simulink model "power_microgrid_v5_battery"  (R2018b)
settings: Solver=ode23tb  StartTime=0.0  StopTime=24*60*60  FixedStep=1/(1000)  MaxStep=60  RelTol=1e-4
PreLoadFcn:
  | load('solar_load_data_24h.mat')
PostLoadFcn:
  | data = xlsread('Domestic_data_all_x3','Sheet1');
  | breakpoints1 = data(2:end,1)'
  | breakpoints2 = data(1,2:end)
  | table_data = data(2:end,2:end)
values from neighbouring files (symbols this model uses):
  SPD_1min = [0 0 0 0 0 0 0 0 0 0 0 0 ... (1441 elements, 1441x1)]    [default_PV_data.mat]
  SPT_1min = [0 60 120 180 240 300 360 420 480 540 600 660 ... (1441 elements, 1441x1)]    [default_PV_data.mat]
libraries: powerlib x155
(part 1 of 5)
Description:
  | Copyright 2008-2018 The MathWorks, Inc.
settings Model: ModifiedByFormat=SPS  ExtModeTrigMode=oneshot  ExtModeArmWhenConnect=off  Creator=MathWorks  LastModifiedBy=SPS
settings SolverCC: InitialStep=1e-4  ZeroCrossAlgorithm=Adaptive
settings DataIOCC: SaveFormat=Array  SignalLoggingSaveFormat=ModelDataLogs  SaveOutput=off  SaveTime=off  SignalLoggingName=sigsOut
settings OptimizationCC: BooleanDataType=off  ExpressionDepthLimit=2147483647  InitFltsAndDblsToZero=on  LifeSpan=inf
settings DebuggingCC: AlgebraicLoopMsg=none  SaveWithParameterizedLinksMsg=none  UnderspecifiedInitializationDetection=Classic  MergeDetectMultiDrivingBlocksExec=none  SignalResolutionControl=TryResolveAllWithWarning  MultiTaskDSMMsg=warning  MultiTaskCondExecSysMsg=none  FcnCallInpInsideContextMsg=warning  AllowSymbolicDim=off  StateNameClashWarn=warning  SFUnexpectedBacktrackingDiag=warning  SFNoUnconditionalDefaultTransitionDiag=warning  SFExecutionAtInitializationDiag=none
settings HardwareCC: ProdBitPerPointer=32  ProdBitPerSizeT=32  ProdBitPerPtrDiffT=32  ProdLargestAtomicFloat=None  ProdIntDivRoundTo=Undefined  ProdEndianess=Unspecified  ProdWordSize=32  ProdHWDeviceType=32-bit Generic  TargetUnknown=on
settings ModelReferenceCC: PropagateSignalLabelsOutOfModel=off
settings SFSimCC: SimUseLocalCustomCode=off
settings RTWCC: Description=Generic Real-Time Target  RTWUseLocalCustomCode=off
settings CodeAppCC: StateflowObjectComments=on
settings GRTTargetCC: TargetFcnLib=ansi_tfl_tmw.mat  TargetLangStandard=C89/C90 (ANSI)  GeneratePreprocessorConditionals=Disable all  CombineOutputUpdateFcns=off  GRTInterface=on
settings ConfigComp: CovMetricSettings=dw  CovHtmlReporting=on  CovSaveCumulativeToWorkspaceVar=on  CovSaveSingleToWorkspaceVar=on  CovExternalEMLEnable=off  CovSFcnEnable=off
settings SimscapeCC: SimscapeNormalizeSystem=off

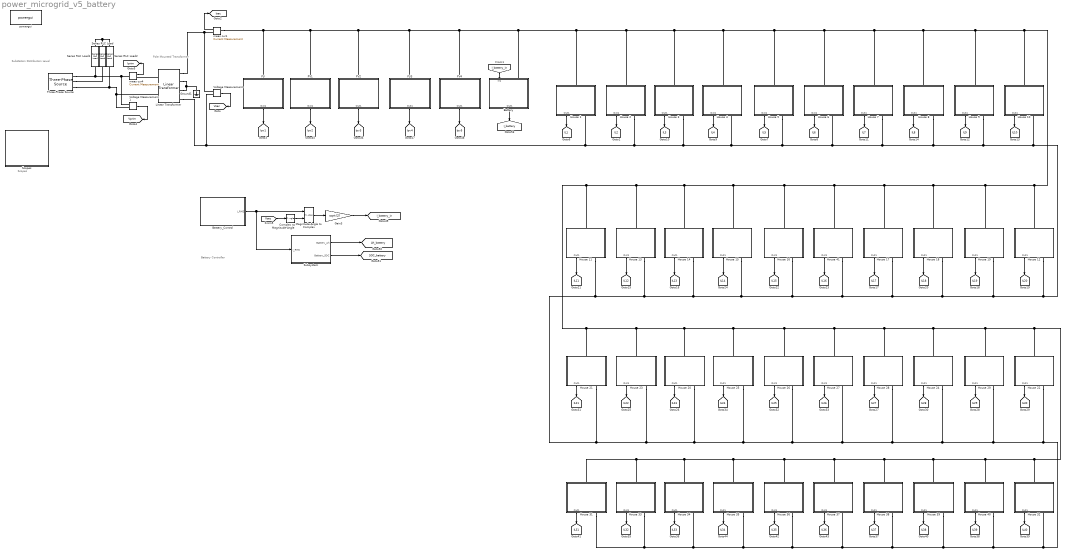
== system power_microgrid_v5_battery ==
  note: Substation Distribution Level
  note: Pole Mounted
      | Transformer
  note: Scopes
  note: Battery Controller
  Battery : Subsystem
  Battery_Control : Subsystem
  Complex to Magnitude-Angle : ComplexToMagnitudeAngle  Output=Angle
  Gain3 : Gain  Gain=sqrt(2)
  Ground1 : powerlib/Elements/Ground  LConnTagsString=a
      settings: SourceProductName=Simscape Electrical
  House 1 : Subsystem
      mask Display: image(imread('house.jpg'))
  House 10 : Subsystem
      mask Display: image(imread('house.jpg'))
  House 11 : Subsystem
      mask Display: image(imread('house.jpg'))
  House 12 : Subsystem
      mask Display: image(imread('house.jpg'))
  House 13 : Subsystem
      mask Display: image(imread('house.jpg'))
  House 14 : Subsystem
      mask Display: image(imread('house.jpg'))
  House 15 : Subsystem
      mask Display: image(imread('house.jpg'))
  House 16 : Subsystem
      mask Display: image(imread('house.jpg'))
  House 17 : Subsystem
      mask Display: image(imread('house.jpg'))
  House 18 : Subsystem
      mask Display: image(imread('house.jpg'))
  House 19 : Subsystem
      mask Display: image(imread('house.jpg'))
  House 2 : Subsystem
      mask Display: image(imread('house.jpg'))
  House 20 : Subsystem
      mask Display: image(imread('house.jpg'))
  House 21 : Subsystem
      mask Display: image(imread('house.jpg'))
  House 22 : Subsystem
      mask Display: image(imread('house.jpg'))
  House 23 : Subsystem
      mask Display: image(imread('house.jpg'))
  House 24 : Subsystem
      mask Display: image(imread('house.jpg'))
  House 25 : Subsystem
      mask Display: image(imread('house.jpg'))
  House 26 : Subsystem
      mask Display: image(imread('house.jpg'))
  House 27 : Subsystem
      mask Display: image(imread('house.jpg'))
  House 28 : Subsystem
      mask Display: image(imread('house.jpg'))
  House 29 : Subsystem
      mask Display: image(imread('house.jpg'))
  House 3 : Subsystem
      mask Display: image(imread('house.jpg'))
  House 31 : Subsystem
      mask Display: image(imread('house.jpg'))
  House 32 : Subsystem
      mask Display: image(imread('house.jpg'))
  House 33 : Subsystem
      mask Display: image(imread('house.jpg'))
  House 34 : Subsystem
      mask Display: image(imread('house.jpg'))
  House 35 : Subsystem
      mask Display: image(imread('house.jpg'))
  House 36 : Subsystem
      mask Display: image(imread('house.jpg'))
  House 37 : Subsystem
      mask Display: image(imread('house.jpg'))
  House 38 : Subsystem
      mask Display: image(imread('house.jpg'))
  House 39 : Subsystem
      mask Display: image(imread('house.jpg'))
  House 4 : Subsystem
      mask Display: image(imread('house.jpg'))
  House 40 : Subsystem
      mask Display: image(imread('house.jpg'))
  House 41 : Subsystem
      mask Display: image(imread('house.jpg'))
  House 5 : Subsystem
      mask Display: image(imread('house.jpg'))
  House 6 : Subsystem
      mask Display: image(imread('house.jpg'))
  House 7 : Subsystem
      mask Display: image(imread('house.jpg'))
  House 8 : Subsystem
      mask Display: image(imread('house.jpg'))
  House 9 : Subsystem
      mask Display: image(imread('house.jpg'))
  Linear Transformer : powerlib/Elements/Linear Transformer  UNITS=SI  NominalPower=[30e3 50]  winding1=[11e3 0 0]  winding2=[115 0 0]  ThreeWindings=on  winding3=[115 0 0]  RmLm=[1e7 1e7]  Measurements=None  DataType=on
      settings: SourceProductName=Simscape Electrical
  Magnitude-Angle to Complex : MagnitudeAngleToComplex
  PV : Subsystem
      mask Display: image(imread('pv.jpg'))
  PV1 : Subsystem
      mask Display: image(imread('pv.jpg'))
  PV2 : Subsystem
      mask Display: image(imread('pv.jpg'))
  PV3 : Subsystem
      mask Display: image(imread('pv.jpg'))
  PV4 : Subsystem
      mask Display: image(imread('pv.jpg'))
  Scopes : Subsystem
      mask Display: image(imread('scope.png'))
  Series RLC Load : powerlib/Elements/Series RLC Load  LConnTagsString=a  RConnTagsString=__new0  NominalVoltage=1000  NominalFrequency=50  ActivePower=10e3  InductivePower=100  CapacitivePower=100  Setx0=off  InitialVoltage=0  SetiL0=off  InitialCurrent=0  Measurements=None  LoadType=constant Z
      settings: SourceProductName=Simscape Electrical
  Series RLC Load1 : powerlib/Elements/Series RLC Load  LConnTagsString=a  RConnTagsString=__new0  NominalVoltage=1000  NominalFrequency=50  ActivePower=100e3  InductivePower=100  CapacitivePower=100  Setx0=off  InitialVoltage=0  SetiL0=off  InitialCurrent=0  Measurements=None  LoadType=constant Z
      settings: SourceProductName=Simscape Electrical
  Series RLC Load2 : powerlib/Elements/Series RLC Load  LConnTagsString=a  RConnTagsString=__new0  NominalVoltage=1000  NominalFrequency=50  ActivePower=10e3  InductivePower=100  CapacitivePower=100  Setx0=off  InitialVoltage=0  SetiL0=off  InitialCurrent=0  Measurements=None  LoadType=constant Z
      settings: SourceProductName=Simscape Electrical
  Subsystem : Subsystem  mask{AH=400}
      mask prompts: AH "Capacity[Ah]"
  Three-Phase Source : powerlib/Electrical Sources/Three-Phase Source  InternalConnection=Yg  VoltagePhases=off  Voltage=11e3  PhaseAngle=0  Voltage_phases=[25e3 25e3 25e3]/sqrt(3)  PhaseAngles_phases=[0 -120 +120]  Frequency=50  NonIdealSource=off  SpecifyImpedance=on  Resistance=0.8929  Inductance=16.58e-3  ShortCircuitLevel=100e6  BaseVoltage=25e3  XRratio=7  BusType=swing  Pref=0  Qref=0  Prefabc=[10e3, 10e3, 10e3]  Qrefabc=[0, 0, 0]  Qmin=-inf  Qmax=inf
      settings: SourceProductName=Simscape Electrical
  Voltage Measurement : powerlib/Measurements/Voltage Measurement  PhasorSimulation=on  OutputType=Complex  PSBequivalent=0
      settings: SourceProductName=Simscape Electrical
  Voltage Measurement1 : powerlib/Measurements/Voltage Measurement  PhasorSimulation=on  OutputType=Complex  PSBequivalent=0
      settings: SourceProductName=Simscape Electrical
  meas cur1 : powerlib/Measurements/Current Measurement  PhasorSimulation=on  OutputType=Complex  PSBequivalent=0
      settings: SourceProductName=Simscape Electrical
  meas cur4 : powerlib/Measurements/Current Measurement  PhasorSimulation=on  OutputType=Complex  PSBequivalent=0
      settings: SourceProductName=Simscape Electrical
  powergui : powerlib/powergui  SimulationMode=Phasor  SampleTime=1/60/100  frequency=50  Iterations=50  frequencyindice=50  Pbase=100e6  ErrMax=1e-4  UnitsV=kV  UnitsW=MW  buscounter=0  FunctionMessages=off  echomessages=off  EnableUseOfTLC=off  CurrentSourceSwitches=off  DisableSnubberDevices=off  DisableRonSwitches=off  DisableVfSwitches=off  DisplayEquations=off  SolverType=Tustin  Interpol=off  ExternalGateDelay=off  methode=off  Ts=0  x0status=blocks  SPID=off  SwTol=0  HookPort=off  RestoreLinks=warning  ResistiveCurrentMeasurement=off  Frange=[0:2:500]  Ylog=off  Xlog=on  ShowGrid=off  save=off  variable=ZData  structure=0  ZoomFFT=on  StartTime=0.0  cycles=1  DisplayStyle=1  fundamental=60  FreqAxis=off  MaxFrequency=1000  frequencyindicesteady=1  RmsSteady=1  display=off
  tag scope: Ah_battery=global, IL10=global, IL11=global, IL12=global, IL13=global, IL14=global, IL15=global, IL16=global, IL17=global, IL18=global, IL19=global, IL1=global, IL20=global, IL21=global, IL22=global, IL23=global, IL24=global, IL25=global, IL26=global, IL27=global, IL28=global, IL29=global, IL2=global, IL30=global, IL31=global, IL32=global, IL33=global, IL34=global, IL35=global, IL36=global, IL37=global, IL38=global, IL39=global, IL3=global, IL40=global, IL4=global, IL5=global, IL6=global, IL7=global, IL8=global, IL9=global, I_battery=global, I_battery_in=global, Iprim=global, Ipv1=global, Ipv2=global, Ipv3=global, Ipv4=global, Ipv5=global, Isec=global, SOC_battery=global, Vprim=global, Vsec=global
  wires:
  House 2/1(Out1) -> [IL2]
  House 1/1(Out1) -> [IL1]
  meas cur1/1 -> [Isec]
  House 3/1(Out1) -> [IL3]
  Voltage Measurement1/1 -> [Vprim]
  meas cur4/1 -> [Iprim]
  Voltage Measurement/1 -> [Vsec]
  House 4/1(Out1) -> [IL4]
  House 5/1(Out1) -> [IL5]
  House 6/1(Out1) -> [IL6]
  PV/1(Out1) -> [Ipv1]
  House 7/1(Out1) -> [IL7]
  House 9/1(Out1) -> [IL9]
  House 10/1(Out1) -> [IL10]
  House 8/1(Out1) -> [IL8]
  House 13/1(Out1) -> [IL12]
  House 17/1(Out1) -> [IL17]
  House 11/1(Out1) -> [IL11]
  House 14/1(Out1) -> [IL13]
  House 15/1(Out1) -> [IL14]
  House 18/1(Out1) -> [IL18]
  House 12/1(Out1) -> [IL20]
  House 19/1(Out1) -> [IL19]
  House 41/1(Out1) -> [IL16]
  House 16/1(Out1) -> [IL15]
  House 28/1(Out1) -> [IL27]
  House 27/1(Out1) -> [IL26]
  House 25/1(Out1) -> [IL24]
  House 26/1(Out1) -> [IL25]
  House 24/1(Out1) -> [IL28]
  House 20/1(Out1) -> [IL23]
  House 23/1(Out1) -> [IL22]
  House 29/1(Out1) -> [IL29]
  House 22/1(Out1) -> [IL30]
  House 21/1(Out1) -> [IL21]
  House 32/1(Out1) -> [IL40]
  House 38/1(Out1) -> [IL37]
  House 39/1(Out1) -> [IL38]
  House 37/1(Out1) -> [IL36]
  House 35/1(Out1) -> [IL34]
  House 36/1(Out1) -> [IL35]
  House 34/1(Out1) -> [IL33]
  House 33/1(Out1) -> [IL32]
  House 40/1(Out1) -> [IL39]
  House 31/1(Out1) -> [IL31]
  PV1/1(Out1) -> [Ipv2]
  PV2/1(Out1) -> [Ipv3]
  PV3/1(Out1) -> [Ipv4]
  PV4/1(Out1) -> [Ipv5]
  [I_battery_in] -> Battery/1(In1)
  Battery/1(Out1) -> [I_battery]
  Gain3/1 -> [I_battery_in]
  Battery_Control/1(I_RMS) -> Subsystem/1(I_RMS), Magnitude-Angle to Complex/1
  Magnitude-Angle to Complex/1 -> Gain3/1
  [Vsec] -> Complex to Magnitude-Angle/1
  Subsystem/1(Battery_Ah) -> [Ah_battery]
  Subsystem/2(Battery_SOC) -> [SOC_battery]
  Complex to Magnitude-Angle/1 -> Magnitude-Angle to Complex/2
  connections:
  Three-Phase Source/RConn1 -- Series RLC Load1/RConn1 -- meas cur4/LConn1 -- Voltage Measurement1/LConn1
  Three-Phase Source/RConn3 -- Series RLC Load2/RConn1 -- Linear Transformer/LConn2 -- Voltage Measurement1/LConn2
  Ground1/LConn1 -- Linear Transformer/RConn2 -- Linear Transformer/RConn3
  Three-Phase Source/RConn2 -- Series RLC Load/RConn1
  Series RLC Load1/LConn1 -- Series RLC Load/LConn1 -- Series RLC Load2/LConn1
  Linear Transformer/LConn1 -- meas cur4/RConn1
  Voltage Measurement/LConn1 -- meas cur1/RConn1 -- Linear Transformer/RConn1
  meas cur1/LConn1 -- PV/LConn1 -- PV1/LConn1 -- PV2/LConn1 -- PV3/LConn1 -- PV4/LConn1 -- Battery/LConn1 -- House 1/LConn1 -- House 2/LConn1 -- House 3/LConn1 -- House 4/LConn1 -- House 5/LConn1 -- House 10/LConn1 -- House 12/LConn1 -- House 19/LConn1 -- House 18/LConn1 -- House 17/LConn1 -- House 41/LConn1 -- House 16/LConn1 -- House 15/LConn1 -- House 14/LConn1 -- House 13/LConn1 -- House 11/LConn1 -- House 21/LConn1 -- House 23/LConn1 -- House 20/LConn1 -- House 24/LConn1 -- House 29/LConn1 -- House 22/LConn1 -- House 32/LConn1 -- House 40/LConn1 -- House 39/LConn1 -- House 38/LConn1 -- House 37/LConn1 -- House 36/LConn1 -- House 35/LConn1 -- House 33/LConn1 -- House 31/LConn1 -- House 34/LConn1 -- House 28/LConn1 -- House 27/LConn1 -- House 26/LConn1 -- House 25/LConn1 -- House 9/LConn1 -- House 8/LConn1 -- House 7/LConn1 -- House 6/LConn1
  House 9/RConn1 -- House 10/RConn1 -- House 12/RConn1 -- House 18/RConn1 -- House 17/RConn1 -- House 16/RConn1 -- House 15/RConn1 -- House 14/RConn1 -- House 11/RConn1 -- House 20/RConn1 -- House 26/RConn1 -- House 29/RConn1 -- House 22/RConn1 -- House 39/RConn1 -- House 38/RConn1 -- House 37/RConn1 -- House 36/RConn1 -- House 35/RConn1 -- House 34/RConn1 -- House 31/RConn1 -- House 33/RConn1 -- House 40/RConn1 -- House 32/RConn1 -- House 24/RConn1 -- House 28/RConn1 -- House 27/RConn1 -- House 25/RConn1 -- House 23/RConn1 -- House 21/RConn1 -- House 13/RConn1 -- House 41/RConn1 -- House 19/RConn1 -- House 8/RConn1 -- House 5/RConn1 -- House 4/RConn1 -- House 3/RConn1 -- House 2/RConn1 -- Linear Transformer/RConn4 -- Voltage Measurement/LConn2 -- House 1/RConn1 -- House 6/RConn1 -- House 7/RConn1

== system power_microgrid_v5_battery/Battery ==
  In1 : Inport
  Controlled Current Source1 : powerlib/Electrical Sources/Controlled Current Source  Initialize=on  Source_Type=AC  Amplitude=0  Phase=0  Frequency=50  Measurements=None
      settings: SourceProductName=Simscape Electrical
  Ground3 : powerlib/Elements/Ground  LConnTagsString=a
      settings: SourceProductName=Simscape Electrical
  Snubber : powerlib/Elements/Series RLC Branch  LConnTagsString=__new0  RConnTagsString=__new0  BranchType=R  Resistance=1e6  Inductance=1e-3  SetiL0=off  InitialCurrent=0  Capacitance=1e-6  Setx0=off  InitialVoltage=0  Measurements=None
      settings: SourceProductName=Simscape Electrical
  meas cur6 : powerlib/Measurements/Current Measurement  PhasorSimulation=on  OutputType=Complex  PSBequivalent=0
      settings: SourceProductName=Simscape Electrical
  Conn1 : PMIOPort  Side=Left
  Out1 : Outport
  wires:
  meas cur6/1 -> Out1/1
  In1/1 -> Controlled Current Source1/1
  connections:
  Controlled Current Source1/LConn1 -- Ground3/LConn1 -- Snubber/RConn1
  Controlled Current Source1/RConn1 -- Snubber/LConn1 -- meas cur6/LConn1
  Conn1/RConn1 -- meas cur6/RConn1

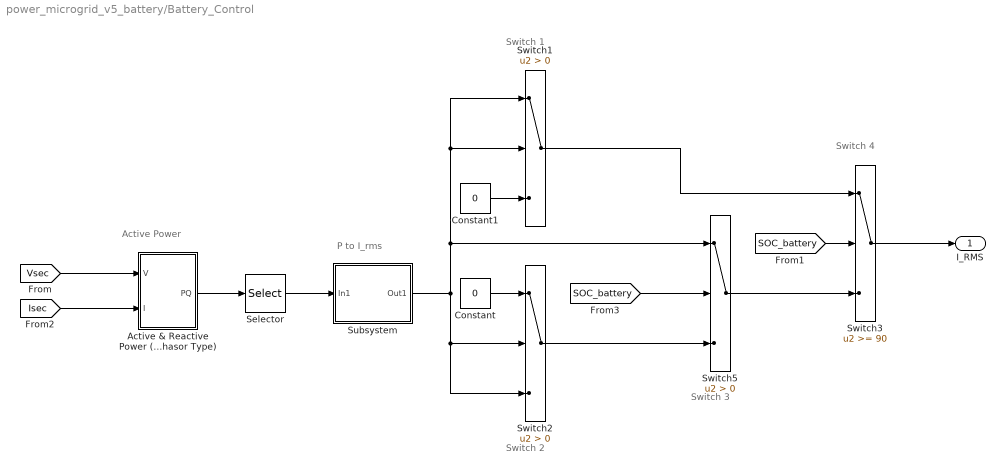
== system power_microgrid_v5_battery/Battery_Control ==
  note: P to I_rms
  note: Switch 4
  note: Switch 3
  note: Switch 2
  note: Switch 1
  note: Active Power
  Active & Reactive Power (Phasor Type) : Subsystem  DialogController=POWERSYS.PowerSysDialog  mask(Active & Reactive Power (Phasor Type)){}
      mask help: Active & Reactive Power (Phasor Type)
      mask init:
      | power_initmask();
      mask Help: This block is part of a subset of blocks in the Extras library that does not have documentation associated with it, other than the block mask description.
      mask Display: disp('')
  Constant : Constant  Value=0
  Constant1 : Constant  Value=0
  Selector : Selector  InputPortWidth=2  IndexOptions=Index vector (dialog)  Indices=1  OutputSizes=1
  Subsystem : Subsystem
  Switch1 : Switch  Criteria=u2 > Threshold
  Switch2 : Switch  Criteria=u2 > Threshold
  Switch3 : Switch  Threshold=90
  Switch5 : Switch  Criteria=u2 > Threshold
  I_RMS : Outport  OutputWhenDisabled=reset  InitialOutput=0
  wires:
  Active & Reactive Power (Phasor Type)/1(PQ) -> Selector/1
  [Isec] -> Active & Reactive Power (Phasor Type)/2(I)
  [Vsec] -> Active & Reactive Power (Phasor Type)/1(V)
  [SOC_battery] -> Switch5/2
  Switch2/1 -> Switch5/3
  Constant/1 -> Switch2/1
  Constant1/1 -> Switch1/3
  Switch1/1 -> Switch3/1
  Switch5/1 -> Switch3/3
  Switch3/1 -> I_RMS/1
  [SOC_battery] -> Switch3/2
  Subsystem/1(Out1) -> Switch2/2, Switch2/3, Switch1/1, Switch1/2, Switch5/1
  Selector/1 -> Subsystem/1(In1)

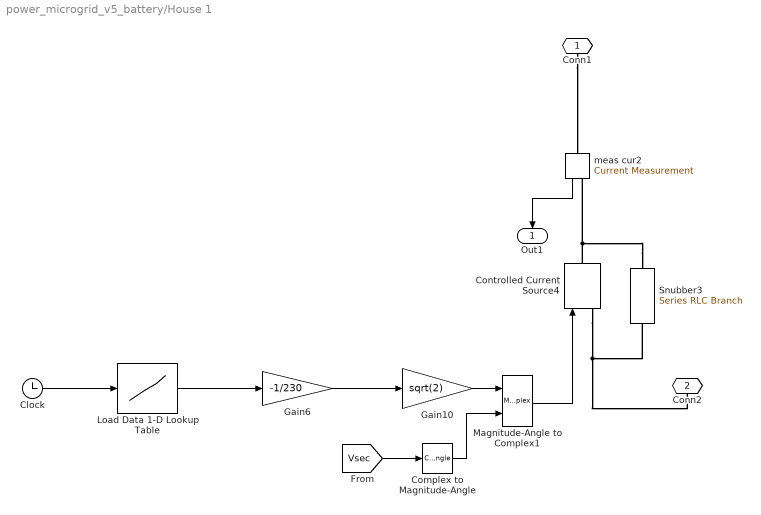
== system power_microgrid_v5_battery/House 1 ==
  Clock : Clock
  Complex to Magnitude-Angle : ComplexToMagnitudeAngle  Output=Angle
  Controlled Current Source4 : powerlib/Electrical Sources/Controlled Current Source  Initialize=on  Source_Type=AC  Amplitude=0  Phase=0  Frequency=50  Measurements=None
      settings: SourceProductName=Simscape Electrical
  Gain10 : Gain  Gain=sqrt(2)
  Gain6 : Gain  Gain=-1/230
  Load Data 1-D Lookup Table : Lookup_n-D  NumberOfTableDimensions=1  BreakpointsForDimension1="[0.00\t600.00\t1200.00\t1800.00\t2400.00\t3000.00\t3600.00\t4200.00\t4800.00\t5400.00\t6000.00\t6600.00\t7200.00\t7800.00\t8400.00\t9000.00\t9600.00\t10200.00\t10800.00\t11400.00\t12000.00\t12600.00\t13200.00\t13800.00\t14400.00\t15000.00\t15600.00\t16200.00\t16800.00\t17400.00\t18000.00\t18600.00\t19200.00\t19800.00\t20400.00\t21000.00\t21600.00\t22200.00\t22800.00\t23400.00\t24000.00\t24600.00\t25200.00\t25800.00\t26400.00\t27000.00\t27600.00\t28200.00\t28800.00\t29400.00\t30000.00\t30600.00\t31200.00\t31800.00\t32400.00\t33000.00\t33600.00\t34200.00\t34800.00\t35400.00\t36000.00\t36600.00\t37200.00\t37800.00\t38400.00\t39000.00\t39600.00\t40200.00\t40800.00\t41400.00\t42000.00\t42600.00\t43200.00\t43800.00\t44400.00\t45000.00\t45600.00\t46200.00\t46800.00\t47400.00\t48000.00\t48600.00\t49200.00\t49800.00\t50400.00\t51000.00\t51600.00\t52200.00\t52800.00\t53400.00\t54000.00\t54600.00\t55200.00\t55800.00\t56400.00\t57000.00\t57600.00\t58200.00\t58800.00\t59400.00\t60000.00\t60600.00\t61200.00\t61800.00\t62400.00\t63000.00\t63600.00\t64200.00\t64800.00\t65400.00\t66000.00\t66600.00\t67200.00\t67800.00\t68400.00\t69000.00\t69600.00\t70200.00\t70800.00\t71400.00\t72000.00\t72600.00\t73200.00\t73800.00\t74400.00\t75000.00\t75600.00\t76200.00\t76800.00\t77400.00\t78000.00\t78600.00\t79200.00\t79800.00\t80400.00\t81000.00\t81600.00\t82200.00\t82800.00\t83400.00\t84000.00\t84600.00\t85200.00\t85800.00\t86400.00]"  BeginIndexSearchUsingPreviousIndexResult=on  Table="[179.5\t163.3\t152.9\t132.5\t118.9\t111.3\t124.6\t103.3\t83.5\t81.2\t85.9\t85.2\t91.9\t95.6\t95.9\t81.8\t83.7\t86.7\t93.8\t81.2\t92.7\t99.4\t112.6\t88.2\t85.6\t78.4\t88.4\t93.9\t86.1\t86.0\t111.7\t143.5\t122.7\t136.8\t142.2\t135.1\t145.6\t141.8\t152.1\t140.3\t167.9\t256.6\t226.1\t263.8\t283.9\t303.3\t279.5\t294.9\t282.3\t288.8\t333.5\t360.9\t421.4\t494.2\t392.5\t439.7\t395.9\t394.4\t364.9\t353.0\t359.1\t370.9\t398.5\t447.4\t344.5\t330.8\t306.8\t331.3\t331.9\t307.6\t371.3\t387.4\t376.6\t360.2\t414.1\t445.1\t411.1\t389.5\t425.2\t340.0\t316.3\t332.8\t352.3\t301.8\t261.8\t298.1\t350.9\t327.8\t296.5\t319.6\t368.4\t327.2\t265.7\t277.9\t292.9\t301.4\t377.9\t336.0\t324.6\t353.8\t389.7\t355.9\t328.4\t325.9\t378.1\t338.0\t379.1\t414.8\t418.1\t464.8\t488.1\t489.1\t485.7\t581.3\t579.7\t526.2\t551.4\t618.6\t628.5\t578.8\t553.3\t481.5\t455.6\t487.9\t507.3\t497.6\t515.4\t510.2\t490.5\t500.5\t494.1\t532.9\t506.5\t466.6\t438.0\t385.4\t381.2\t385.9\t351.7\t371.3\t340.8\t320.2\t277.0\t228.9\t179.5]"  InternalRulePriority=Speed  RndMeth=Simplest  InputSameDT=on
  Magnitude-Angle to Complex1 : MagnitudeAngleToComplex
  Snubber3 : powerlib/Elements/Series RLC Branch  LConnTagsString=__new0  RConnTagsString=__new0  BranchType=R  Resistance=1e6  Inductance=1e-3  SetiL0=off  InitialCurrent=0  Capacitance=1e-6  Setx0=off  InitialVoltage=0  Measurements=None
      settings: SourceProductName=Simscape Electrical
  meas cur2 : powerlib/Measurements/Current Measurement  PhasorSimulation=on  OutputType=Complex  PSBequivalent=0
      settings: SourceProductName=Simscape Electrical
  Conn1 : PMIOPort  Side=Left
  Conn2 : PMIOPort  Port=2  Side=Right
  Out1 : Outport
  wires:
  meas cur2/1 -> Out1/1
  Clock/1 -> Load Data 1-D Lookup Table/1
  Magnitude-Angle to Complex1/1 -> Controlled Current Source4/1
  Load Data 1-D Lookup Table/1 -> Gain6/1
  Complex to Magnitude-Angle/1 -> Magnitude-Angle to Complex1/2
  Gain10/1 -> Magnitude-Angle to Complex1/1
  Gain6/1 -> Gain10/1
  [Vsec] -> Complex to Magnitude-Angle/1
  connections:
  Conn1/RConn1 -- meas cur2/LConn1
  Snubber3/LConn1 -- meas cur2/RConn1 -- Controlled Current Source4/RConn1
  Snubber3/RConn1 -- Controlled Current Source4/LConn1 -- Conn2/RConn1

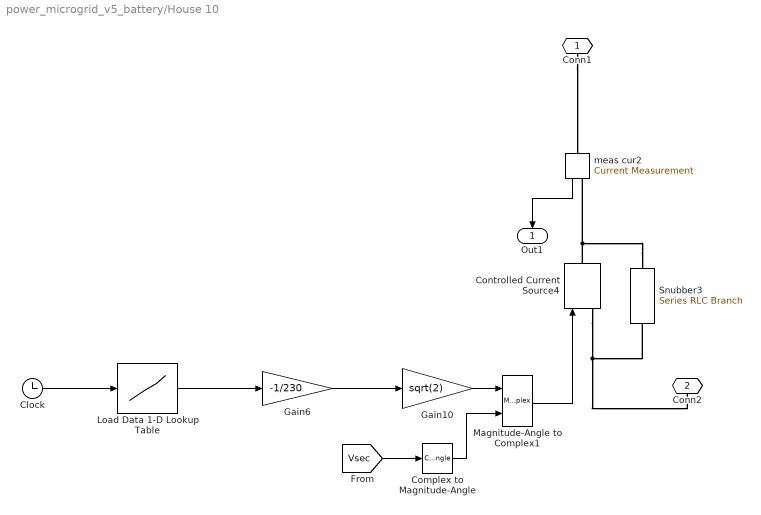
== system power_microgrid_v5_battery/House 10 ==
  Clock : Clock
  Complex to Magnitude-Angle : ComplexToMagnitudeAngle  Output=Angle
  Controlled Current Source4 : powerlib/Electrical Sources/Controlled Current Source  Initialize=on  Source_Type=AC  Amplitude=0  Phase=0  Frequency=50  Measurements=None
      settings: SourceProductName=Simscape Electrical
  Gain10 : Gain  Gain=sqrt(2)
  Gain6 : Gain  Gain=-1/230
  Load Data 1-D Lookup Table : Lookup_n-D  NumberOfTableDimensions=1  BreakpointsForDimension1="[0.00\t600.00\t1200.00\t1800.00\t2400.00\t3000.00\t3600.00\t4200.00\t4800.00\t5400.00\t6000.00\t6600.00\t7200.00\t7800.00\t8400.00\t9000.00\t9600.00\t10200.00\t10800.00\t11400.00\t12000.00\t12600.00\t13200.00\t13800.00\t14400.00\t15000.00\t15600.00\t16200.00\t16800.00\t17400.00\t18000.00\t18600.00\t19200.00\t19800.00\t20400.00\t21000.00\t21600.00\t22200.00\t22800.00\t23400.00\t24000.00\t24600.00\t25200.00\t25800.00\t26400.00\t27000.00\t27600.00\t28200.00\t28800.00\t29400.00\t30000.00\t30600.00\t31200.00\t31800.00\t32400.00\t33000.00\t33600.00\t34200.00\t34800.00\t35400.00\t36000.00\t36600.00\t37200.00\t37800.00\t38400.00\t39000.00\t39600.00\t40200.00\t40800.00\t41400.00\t42000.00\t42600.00\t43200.00\t43800.00\t44400.00\t45000.00\t45600.00\t46200.00\t46800.00\t47400.00\t48000.00\t48600.00\t49200.00\t49800.00\t50400.00\t51000.00\t51600.00\t52200.00\t52800.00\t53400.00\t54000.00\t54600.00\t55200.00\t55800.00\t56400.00\t57000.00\t57600.00\t58200.00\t58800.00\t59400.00\t60000.00\t60600.00\t61200.00\t61800.00\t62400.00\t63000.00\t63600.00\t64200.00\t64800.00\t65400.00\t66000.00\t66600.00\t67200.00\t67800.00\t68400.00\t69000.00\t69600.00\t70200.00\t70800.00\t71400.00\t72000.00\t72600.00\t73200.00\t73800.00\t74400.00\t75000.00\t75600.00\t76200.00\t76800.00\t77400.00\t78000.00\t78600.00\t79200.00\t79800.00\t80400.00\t81000.00\t81600.00\t82200.00\t82800.00\t83400.00\t84000.00\t84600.00\t85200.00\t85800.00\t86400.00]"  BeginIndexSearchUsingPreviousIndexResult=on  Table="[179.5\t163.3\t152.9\t132.5\t118.9\t111.3\t124.6\t103.3\t83.5\t81.2\t85.9\t85.2\t91.9\t95.6\t95.9\t81.8\t83.7\t86.7\t93.8\t81.2\t92.7\t99.4\t112.6\t88.2\t85.6\t78.4\t88.4\t93.9\t86.1\t86.0\t111.7\t143.5\t122.7\t136.8\t142.2\t135.1\t145.6\t141.8\t152.1\t140.3\t167.9\t256.6\t226.1\t263.8\t283.9\t303.3\t279.5\t294.9\t282.3\t288.8\t333.5\t360.9\t421.4\t494.2\t392.5\t439.7\t395.9\t394.4\t364.9\t353.0\t359.1\t370.9\t398.5\t447.4\t344.5\t330.8\t306.8\t331.3\t331.9\t307.6\t371.3\t387.4\t376.6\t360.2\t414.1\t445.1\t411.1\t389.5\t425.2\t340.0\t316.3\t332.8\t352.3\t301.8\t261.8\t298.1\t350.9\t327.8\t296.5\t319.6\t368.4\t327.2\t265.7\t277.9\t292.9\t301.4\t377.9\t336.0\t324.6\t353.8\t389.7\t355.9\t328.4\t325.9\t378.1\t338.0\t379.1\t414.8\t418.1\t464.8\t488.1\t489.1\t485.7\t581.3\t579.7\t526.2\t551.4\t618.6\t628.5\t578.8\t553.3\t481.5\t455.6\t487.9\t507.3\t497.6\t515.4\t510.2\t490.5\t500.5\t494.1\t532.9\t506.5\t466.6\t438.0\t385.4\t381.2\t385.9\t351.7\t371.3\t340.8\t320.2\t277.0\t228.9\t179.5]"  InternalRulePriority=Speed  RndMeth=Simplest  InputSameDT=on
  Magnitude-Angle to Complex1 : MagnitudeAngleToComplex
  Snubber3 : powerlib/Elements/Series RLC Branch  LConnTagsString=__new0  RConnTagsString=__new0  BranchType=R  Resistance=1e6  Inductance=1e-3  SetiL0=off  InitialCurrent=0  Capacitance=1e-6  Setx0=off  InitialVoltage=0  Measurements=None
      settings: SourceProductName=Simscape Electrical
  meas cur2 : powerlib/Measurements/Current Measurement  PhasorSimulation=on  OutputType=Complex  PSBequivalent=0
      settings: SourceProductName=Simscape Electrical
  Conn1 : PMIOPort  Side=Left
  Conn2 : PMIOPort  Port=2  Side=Right
  Out1 : Outport
  wires:
  meas cur2/1 -> Out1/1
  Clock/1 -> Load Data 1-D Lookup Table/1
  Magnitude-Angle to Complex1/1 -> Controlled Current Source4/1
  Load Data 1-D Lookup Table/1 -> Gain6/1
  Complex to Magnitude-Angle/1 -> Magnitude-Angle to Complex1/2
  Gain10/1 -> Magnitude-Angle to Complex1/1
  Gain6/1 -> Gain10/1
  [Vsec] -> Complex to Magnitude-Angle/1
  connections:
  Conn1/RConn1 -- meas cur2/LConn1
  Snubber3/LConn1 -- meas cur2/RConn1 -- Controlled Current Source4/RConn1
  Snubber3/RConn1 -- Controlled Current Source4/LConn1 -- Conn2/RConn1

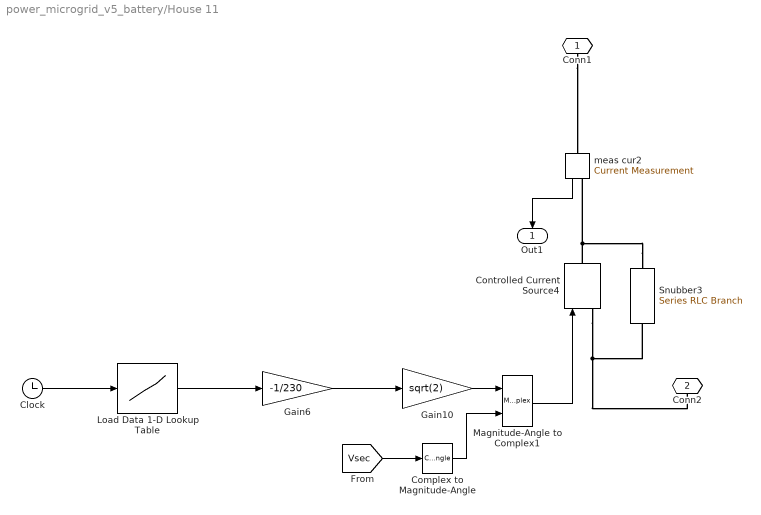
== system power_microgrid_v5_battery/House 11 ==
  Clock : Clock
  Complex to Magnitude-Angle : ComplexToMagnitudeAngle  Output=Angle
  Controlled Current Source4 : powerlib/Electrical Sources/Controlled Current Source  Initialize=on  Source_Type=AC  Amplitude=0  Phase=0  Frequency=50  Measurements=None
      settings: SourceProductName=Simscape Electrical
  Gain10 : Gain  Gain=sqrt(2)
  Gain6 : Gain  Gain=-1/230
  Load Data 1-D Lookup Table : Lookup_n-D  NumberOfTableDimensions=1  BreakpointsForDimension1="[0.00\t600.00\t1200.00\t1800.00\t2400.00\t3000.00\t3600.00\t4200.00\t4800.00\t5400.00\t6000.00\t6600.00\t7200.00\t7800.00\t8400.00\t9000.00\t9600.00\t10200.00\t10800.00\t11400.00\t12000.00\t12600.00\t13200.00\t13800.00\t14400.00\t15000.00\t15600.00\t16200.00\t16800.00\t17400.00\t18000.00\t18600.00\t19200.00\t19800.00\t20400.00\t21000.00\t21600.00\t22200.00\t22800.00\t23400.00\t24000.00\t24600.00\t25200.00\t25800.00\t26400.00\t27000.00\t27600.00\t28200.00\t28800.00\t29400.00\t30000.00\t30600.00\t31200.00\t31800.00\t32400.00\t33000.00\t33600.00\t34200.00\t34800.00\t35400.00\t36000.00\t36600.00\t37200.00\t37800.00\t38400.00\t39000.00\t39600.00\t40200.00\t40800.00\t41400.00\t42000.00\t42600.00\t43200.00\t43800.00\t44400.00\t45000.00\t45600.00\t46200.00\t46800.00\t47400.00\t48000.00\t48600.00\t49200.00\t49800.00\t50400.00\t51000.00\t51600.00\t52200.00\t52800.00\t53400.00\t54000.00\t54600.00\t55200.00\t55800.00\t56400.00\t57000.00\t57600.00\t58200.00\t58800.00\t59400.00\t60000.00\t60600.00\t61200.00\t61800.00\t62400.00\t63000.00\t63600.00\t64200.00\t64800.00\t65400.00\t66000.00\t66600.00\t67200.00\t67800.00\t68400.00\t69000.00\t69600.00\t70200.00\t70800.00\t71400.00\t72000.00\t72600.00\t73200.00\t73800.00\t74400.00\t75000.00\t75600.00\t76200.00\t76800.00\t77400.00\t78000.00\t78600.00\t79200.00\t79800.00\t80400.00\t81000.00\t81600.00\t82200.00\t82800.00\t83400.00\t84000.00\t84600.00\t85200.00\t85800.00\t86400.00]"  BeginIndexSearchUsingPreviousIndexResult=on  Table="[179.5\t163.3\t152.9\t132.5\t118.9\t111.3\t124.6\t103.3\t83.5\t81.2\t85.9\t85.2\t91.9\t95.6\t95.9\t81.8\t83.7\t86.7\t93.8\t81.2\t92.7\t99.4\t112.6\t88.2\t85.6\t78.4\t88.4\t93.9\t86.1\t86.0\t111.7\t143.5\t122.7\t136.8\t142.2\t135.1\t145.6\t141.8\t152.1\t140.3\t167.9\t256.6\t226.1\t263.8\t283.9\t303.3\t279.5\t294.9\t282.3\t288.8\t333.5\t360.9\t421.4\t494.2\t392.5\t439.7\t395.9\t394.4\t364.9\t353.0\t359.1\t370.9\t398.5\t447.4\t344.5\t330.8\t306.8\t331.3\t331.9\t307.6\t371.3\t387.4\t376.6\t360.2\t414.1\t445.1\t411.1\t389.5\t425.2\t340.0\t316.3\t332.8\t352.3\t301.8\t261.8\t298.1\t350.9\t327.8\t296.5\t319.6\t368.4\t327.2\t265.7\t277.9\t292.9\t301.4\t377.9\t336.0\t324.6\t353.8\t389.7\t355.9\t328.4\t325.9\t378.1\t338.0\t379.1\t414.8\t418.1\t464.8\t488.1\t489.1\t485.7\t581.3\t579.7\t526.2\t551.4\t618.6\t628.5\t578.8\t553.3\t481.5\t455.6\t487.9\t507.3\t497.6\t515.4\t510.2\t490.5\t500.5\t494.1\t532.9\t506.5\t466.6\t438.0\t385.4\t381.2\t385.9\t351.7\t371.3\t340.8\t320.2\t277.0\t228.9\t179.5]"  InternalRulePriority=Speed  RndMeth=Simplest  InputSameDT=on
  Magnitude-Angle to Complex1 : MagnitudeAngleToComplex
  Snubber3 : powerlib/Elements/Series RLC Branch  LConnTagsString=__new0  RConnTagsString=__new0  BranchType=R  Resistance=1e6  Inductance=1e-3  SetiL0=off  InitialCurrent=0  Capacitance=1e-6  Setx0=off  InitialVoltage=0  Measurements=None
      settings: SourceProductName=Simscape Electrical
  meas cur2 : powerlib/Measurements/Current Measurement  PhasorSimulation=on  OutputType=Complex  PSBequivalent=0
      settings: SourceProductName=Simscape Electrical
  Conn1 : PMIOPort  Side=Left
  Conn2 : PMIOPort  Port=2  Side=Right
  Out1 : Outport
  wires:
  meas cur2/1 -> Out1/1
  Clock/1 -> Load Data 1-D Lookup Table/1
  Magnitude-Angle to Complex1/1 -> Controlled Current Source4/1
  Load Data 1-D Lookup Table/1 -> Gain6/1
  Complex to Magnitude-Angle/1 -> Magnitude-Angle to Complex1/2
  Gain10/1 -> Magnitude-Angle to Complex1/1
  Gain6/1 -> Gain10/1
  [Vsec] -> Complex to Magnitude-Angle/1
  connections:
  Conn1/RConn1 -- meas cur2/LConn1
  Snubber3/LConn1 -- meas cur2/RConn1 -- Controlled Current Source4/RConn1
  Snubber3/RConn1 -- Controlled Current Source4/LConn1 -- Conn2/RConn1

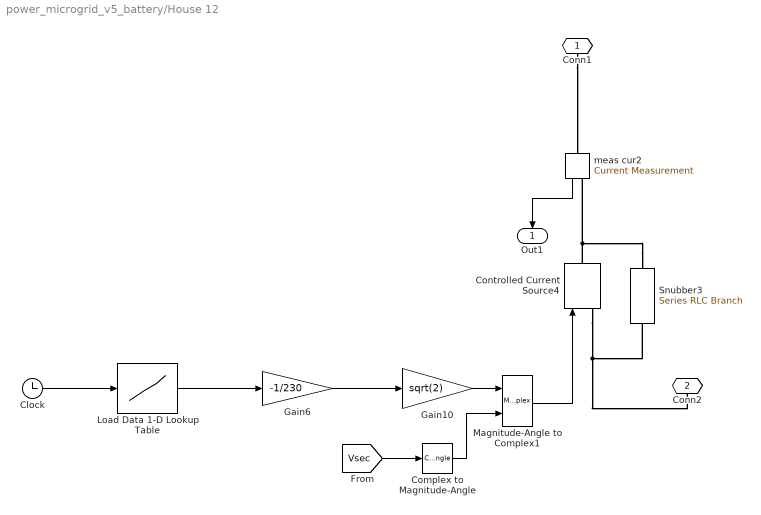
== system power_microgrid_v5_battery/House 12 ==
  Clock : Clock
  Complex to Magnitude-Angle : ComplexToMagnitudeAngle  Output=Angle
  Controlled Current Source4 : powerlib/Electrical Sources/Controlled Current Source  Initialize=on  Source_Type=AC  Amplitude=0  Phase=0  Frequency=50  Measurements=None
      settings: SourceProductName=Simscape Electrical
  Gain10 : Gain  Gain=sqrt(2)
  Gain6 : Gain  Gain=-1/230
  Load Data 1-D Lookup Table : Lookup_n-D  NumberOfTableDimensions=1  BreakpointsForDimension1="[0.00\t600.00\t1200.00\t1800.00\t2400.00\t3000.00\t3600.00\t4200.00\t4800.00\t5400.00\t6000.00\t6600.00\t7200.00\t7800.00\t8400.00\t9000.00\t9600.00\t10200.00\t10800.00\t11400.00\t12000.00\t12600.00\t13200.00\t13800.00\t14400.00\t15000.00\t15600.00\t16200.00\t16800.00\t17400.00\t18000.00\t18600.00\t19200.00\t19800.00\t20400.00\t21000.00\t21600.00\t22200.00\t22800.00\t23400.00\t24000.00\t24600.00\t25200.00\t25800.00\t26400.00\t27000.00\t27600.00\t28200.00\t28800.00\t29400.00\t30000.00\t30600.00\t31200.00\t31800.00\t32400.00\t33000.00\t33600.00\t34200.00\t34800.00\t35400.00\t36000.00\t36600.00\t37200.00\t37800.00\t38400.00\t39000.00\t39600.00\t40200.00\t40800.00\t41400.00\t42000.00\t42600.00\t43200.00\t43800.00\t44400.00\t45000.00\t45600.00\t46200.00\t46800.00\t47400.00\t48000.00\t48600.00\t49200.00\t49800.00\t50400.00\t51000.00\t51600.00\t52200.00\t52800.00\t53400.00\t54000.00\t54600.00\t55200.00\t55800.00\t56400.00\t57000.00\t57600.00\t58200.00\t58800.00\t59400.00\t60000.00\t60600.00\t61200.00\t61800.00\t62400.00\t63000.00\t63600.00\t64200.00\t64800.00\t65400.00\t66000.00\t66600.00\t67200.00\t67800.00\t68400.00\t69000.00\t69600.00\t70200.00\t70800.00\t71400.00\t72000.00\t72600.00\t73200.00\t73800.00\t74400.00\t75000.00\t75600.00\t76200.00\t76800.00\t77400.00\t78000.00\t78600.00\t79200.00\t79800.00\t80400.00\t81000.00\t81600.00\t82200.00\t82800.00\t83400.00\t84000.00\t84600.00\t85200.00\t85800.00\t86400.00]"  BeginIndexSearchUsingPreviousIndexResult=on  Table="[179.5\t163.3\t152.9\t132.5\t118.9\t111.3\t124.6\t103.3\t83.5\t81.2\t85.9\t85.2\t91.9\t95.6\t95.9\t81.8\t83.7\t86.7\t93.8\t81.2\t92.7\t99.4\t112.6\t88.2\t85.6\t78.4\t88.4\t93.9\t86.1\t86.0\t111.7\t143.5\t122.7\t136.8\t142.2\t135.1\t145.6\t141.8\t152.1\t140.3\t167.9\t256.6\t226.1\t263.8\t283.9\t303.3\t279.5\t294.9\t282.3\t288.8\t333.5\t360.9\t421.4\t494.2\t392.5\t439.7\t395.9\t394.4\t364.9\t353.0\t359.1\t370.9\t398.5\t447.4\t344.5\t330.8\t306.8\t331.3\t331.9\t307.6\t371.3\t387.4\t376.6\t360.2\t414.1\t445.1\t411.1\t389.5\t425.2\t340.0\t316.3\t332.8\t352.3\t301.8\t261.8\t298.1\t350.9\t327.8\t296.5\t319.6\t368.4\t327.2\t265.7\t277.9\t292.9\t301.4\t377.9\t336.0\t324.6\t353.8\t389.7\t355.9\t328.4\t325.9\t378.1\t338.0\t379.1\t414.8\t418.1\t464.8\t488.1\t489.1\t485.7\t581.3\t579.7\t526.2\t551.4\t618.6\t628.5\t578.8\t553.3\t481.5\t455.6\t487.9\t507.3\t497.6\t515.4\t510.2\t490.5\t500.5\t494.1\t532.9\t506.5\t466.6\t438.0\t385.4\t381.2\t385.9\t351.7\t371.3\t340.8\t320.2\t277.0\t228.9\t179.5]"  InternalRulePriority=Speed  RndMeth=Simplest  InputSameDT=on
  Magnitude-Angle to Complex1 : MagnitudeAngleToComplex
  Snubber3 : powerlib/Elements/Series RLC Branch  LConnTagsString=__new0  RConnTagsString=__new0  BranchType=R  Resistance=1e6  Inductance=1e-3  SetiL0=off  InitialCurrent=0  Capacitance=1e-6  Setx0=off  InitialVoltage=0  Measurements=None
      settings: SourceProductName=Simscape Electrical
  meas cur2 : powerlib/Measurements/Current Measurement  PhasorSimulation=on  OutputType=Complex  PSBequivalent=0
      settings: SourceProductName=Simscape Electrical
  Conn1 : PMIOPort  Side=Left
  Conn2 : PMIOPort  Port=2  Side=Right
  Out1 : Outport
  wires:
  meas cur2/1 -> Out1/1
  Clock/1 -> Load Data 1-D Lookup Table/1
  Magnitude-Angle to Complex1/1 -> Controlled Current Source4/1
  Load Data 1-D Lookup Table/1 -> Gain6/1
  Complex to Magnitude-Angle/1 -> Magnitude-Angle to Complex1/2
  Gain10/1 -> Magnitude-Angle to Complex1/1
  Gain6/1 -> Gain10/1
  [Vsec] -> Complex to Magnitude-Angle/1
  connections:
  Conn1/RConn1 -- meas cur2/LConn1
  Snubber3/LConn1 -- meas cur2/RConn1 -- Controlled Current Source4/RConn1
  Snubber3/RConn1 -- Controlled Current Source4/LConn1 -- Conn2/RConn1

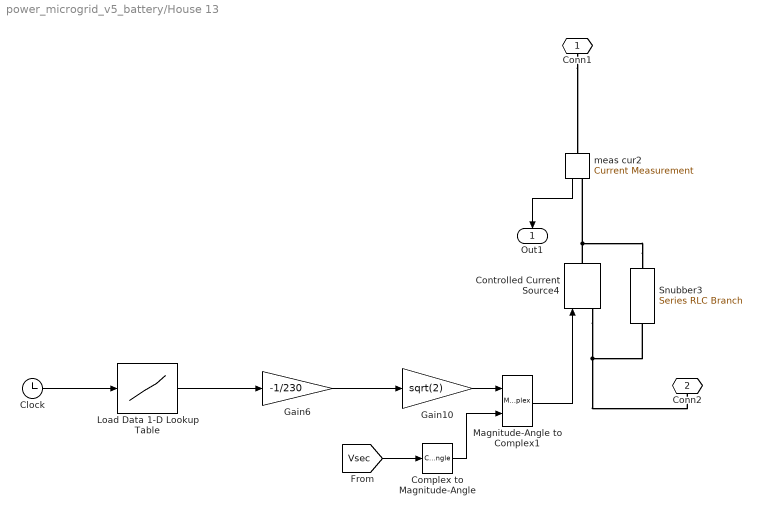
== system power_microgrid_v5_battery/House 13 ==
  Clock : Clock
  Complex to Magnitude-Angle : ComplexToMagnitudeAngle  Output=Angle
  Controlled Current Source4 : powerlib/Electrical Sources/Controlled Current Source  Initialize=on  Source_Type=AC  Amplitude=0  Phase=0  Frequency=50  Measurements=None
      settings: SourceProductName=Simscape Electrical
  Gain10 : Gain  Gain=sqrt(2)
  Gain6 : Gain  Gain=-1/230
  Load Data 1-D Lookup Table : Lookup_n-D  NumberOfTableDimensions=1  BreakpointsForDimension1="[0.00\t600.00\t1200.00\t1800.00\t2400.00\t3000.00\t3600.00\t4200.00\t4800.00\t5400.00\t6000.00\t6600.00\t7200.00\t7800.00\t8400.00\t9000.00\t9600.00\t10200.00\t10800.00\t11400.00\t12000.00\t12600.00\t13200.00\t13800.00\t14400.00\t15000.00\t15600.00\t16200.00\t16800.00\t17400.00\t18000.00\t18600.00\t19200.00\t19800.00\t20400.00\t21000.00\t21600.00\t22200.00\t22800.00\t23400.00\t24000.00\t24600.00\t25200.00\t25800.00\t26400.00\t27000.00\t27600.00\t28200.00\t28800.00\t29400.00\t30000.00\t30600.00\t31200.00\t31800.00\t32400.00\t33000.00\t33600.00\t34200.00\t34800.00\t35400.00\t36000.00\t36600.00\t37200.00\t37800.00\t38400.00\t39000.00\t39600.00\t40200.00\t40800.00\t41400.00\t42000.00\t42600.00\t43200.00\t43800.00\t44400.00\t45000.00\t45600.00\t46200.00\t46800.00\t47400.00\t48000.00\t48600.00\t49200.00\t49800.00\t50400.00\t51000.00\t51600.00\t52200.00\t52800.00\t53400.00\t54000.00\t54600.00\t55200.00\t55800.00\t56400.00\t57000.00\t57600.00\t58200.00\t58800.00\t59400.00\t60000.00\t60600.00\t61200.00\t61800.00\t62400.00\t63000.00\t63600.00\t64200.00\t64800.00\t65400.00\t66000.00\t66600.00\t67200.00\t67800.00\t68400.00\t69000.00\t69600.00\t70200.00\t70800.00\t71400.00\t72000.00\t72600.00\t73200.00\t73800.00\t74400.00\t75000.00\t75600.00\t76200.00\t76800.00\t77400.00\t78000.00\t78600.00\t79200.00\t79800.00\t80400.00\t81000.00\t81600.00\t82200.00\t82800.00\t83400.00\t84000.00\t84600.00\t85200.00\t85800.00\t86400.00]"  BeginIndexSearchUsingPreviousIndexResult=on  Table="[179.5\t163.3\t152.9\t132.5\t118.9\t111.3\t124.6\t103.3\t83.5\t81.2\t85.9\t85.2\t91.9\t95.6\t95.9\t81.8\t83.7\t86.7\t93.8\t81.2\t92.7\t99.4\t112.6\t88.2\t85.6\t78.4\t88.4\t93.9\t86.1\t86.0\t111.7\t143.5\t122.7\t136.8\t142.2\t135.1\t145.6\t141.8\t152.1\t140.3\t167.9\t256.6\t226.1\t263.8\t283.9\t303.3\t279.5\t294.9\t282.3\t288.8\t333.5\t360.9\t421.4\t494.2\t392.5\t439.7\t395.9\t394.4\t364.9\t353.0\t359.1\t370.9\t398.5\t447.4\t344.5\t330.8\t306.8\t331.3\t331.9\t307.6\t371.3\t387.4\t376.6\t360.2\t414.1\t445.1\t411.1\t389.5\t425.2\t340.0\t316.3\t332.8\t352.3\t301.8\t261.8\t298.1\t350.9\t327.8\t296.5\t319.6\t368.4\t327.2\t265.7\t277.9\t292.9\t301.4\t377.9\t336.0\t324.6\t353.8\t389.7\t355.9\t328.4\t325.9\t378.1\t338.0\t379.1\t414.8\t418.1\t464.8\t488.1\t489.1\t485.7\t581.3\t579.7\t526.2\t551.4\t618.6\t628.5\t578.8\t553.3\t481.5\t455.6\t487.9\t507.3\t497.6\t515.4\t510.2\t490.5\t500.5\t494.1\t532.9\t506.5\t466.6\t438.0\t385.4\t381.2\t385.9\t351.7\t371.3\t340.8\t320.2\t277.0\t228.9\t179.5]"  InternalRulePriority=Speed  RndMeth=Simplest  InputSameDT=on
  Magnitude-Angle to Complex1 : MagnitudeAngleToComplex
  Snubber3 : powerlib/Elements/Series RLC Branch  LConnTagsString=__new0  RConnTagsString=__new0  BranchType=R  Resistance=1e6  Inductance=1e-3  SetiL0=off  InitialCurrent=0  Capacitance=1e-6  Setx0=off  InitialVoltage=0  Measurements=None
      settings: SourceProductName=Simscape Electrical
  meas cur2 : powerlib/Measurements/Current Measurement  PhasorSimulation=on  OutputType=Complex  PSBequivalent=0
      settings: SourceProductName=Simscape Electrical
  Conn1 : PMIOPort  Side=Left
  Conn2 : PMIOPort  Port=2  Side=Right
  Out1 : Outport
  wires:
  meas cur2/1 -> Out1/1
  Clock/1 -> Load Data 1-D Lookup Table/1
  Magnitude-Angle to Complex1/1 -> Controlled Current Source4/1
  Load Data 1-D Lookup Table/1 -> Gain6/1
  Complex to Magnitude-Angle/1 -> Magnitude-Angle to Complex1/2
  Gain10/1 -> Magnitude-Angle to Complex1/1
  Gain6/1 -> Gain10/1
  [Vsec] -> Complex to Magnitude-Angle/1
  connections:
  Conn1/RConn1 -- meas cur2/LConn1
  Snubber3/LConn1 -- meas cur2/RConn1 -- Controlled Current Source4/RConn1
  Snubber3/RConn1 -- Controlled Current Source4/LConn1 -- Conn2/RConn1

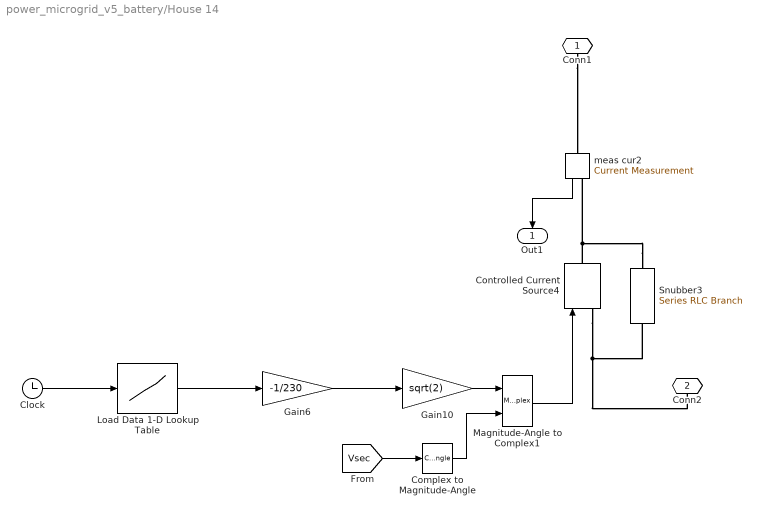
== system power_microgrid_v5_battery/House 14 ==
  Clock : Clock
  Complex to Magnitude-Angle : ComplexToMagnitudeAngle  Output=Angle
  Controlled Current Source4 : powerlib/Electrical Sources/Controlled Current Source  Initialize=on  Source_Type=AC  Amplitude=0  Phase=0  Frequency=50  Measurements=None
      settings: SourceProductName=Simscape Electrical
  Gain10 : Gain  Gain=sqrt(2)
  Gain6 : Gain  Gain=-1/230
  Load Data 1-D Lookup Table : Lookup_n-D  NumberOfTableDimensions=1  BreakpointsForDimension1="[0.00\t600.00\t1200.00\t1800.00\t2400.00\t3000.00\t3600.00\t4200.00\t4800.00\t5400.00\t6000.00\t6600.00\t7200.00\t7800.00\t8400.00\t9000.00\t9600.00\t10200.00\t10800.00\t11400.00\t12000.00\t12600.00\t13200.00\t13800.00\t14400.00\t15000.00\t15600.00\t16200.00\t16800.00\t17400.00\t18000.00\t18600.00\t19200.00\t19800.00\t20400.00\t21000.00\t21600.00\t22200.00\t22800.00\t23400.00\t24000.00\t24600.00\t25200.00\t25800.00\t26400.00\t27000.00\t27600.00\t28200.00\t28800.00\t29400.00\t30000.00\t30600.00\t31200.00\t31800.00\t32400.00\t33000.00\t33600.00\t34200.00\t34800.00\t35400.00\t36000.00\t36600.00\t37200.00\t37800.00\t38400.00\t39000.00\t39600.00\t40200.00\t40800.00\t41400.00\t42000.00\t42600.00\t43200.00\t43800.00\t44400.00\t45000.00\t45600.00\t46200.00\t46800.00\t47400.00\t48000.00\t48600.00\t49200.00\t49800.00\t50400.00\t51000.00\t51600.00\t52200.00\t52800.00\t53400.00\t54000.00\t54600.00\t55200.00\t55800.00\t56400.00\t57000.00\t57600.00\t58200.00\t58800.00\t59400.00\t60000.00\t60600.00\t61200.00\t61800.00\t62400.00\t63000.00\t63600.00\t64200.00\t64800.00\t65400.00\t66000.00\t66600.00\t67200.00\t67800.00\t68400.00\t69000.00\t69600.00\t70200.00\t70800.00\t71400.00\t72000.00\t72600.00\t73200.00\t73800.00\t74400.00\t75000.00\t75600.00\t76200.00\t76800.00\t77400.00\t78000.00\t78600.00\t79200.00\t79800.00\t80400.00\t81000.00\t81600.00\t82200.00\t82800.00\t83400.00\t84000.00\t84600.00\t85200.00\t85800.00\t86400.00]"  BeginIndexSearchUsingPreviousIndexResult=on  Table="[179.5\t163.3\t152.9\t132.5\t118.9\t111.3\t124.6\t103.3\t83.5\t81.2\t85.9\t85.2\t91.9\t95.6\t95.9\t81.8\t83.7\t86.7\t93.8\t81.2\t92.7\t99.4\t112.6\t88.2\t85.6\t78.4\t88.4\t93.9\t86.1\t86.0\t111.7\t143.5\t122.7\t136.8\t142.2\t135.1\t145.6\t141.8\t152.1\t140.3\t167.9\t256.6\t226.1\t263.8\t283.9\t303.3\t279.5\t294.9\t282.3\t288.8\t333.5\t360.9\t421.4\t494.2\t392.5\t439.7\t395.9\t394.4\t364.9\t353.0\t359.1\t370.9\t398.5\t447.4\t344.5\t330.8\t306.8\t331.3\t331.9\t307.6\t371.3\t387.4\t376.6\t360.2\t414.1\t445.1\t411.1\t389.5\t425.2\t340.0\t316.3\t332.8\t352.3\t301.8\t261.8\t298.1\t350.9\t327.8\t296.5\t319.6\t368.4\t327.2\t265.7\t277.9\t292.9\t301.4\t377.9\t336.0\t324.6\t353.8\t389.7\t355.9\t328.4\t325.9\t378.1\t338.0\t379.1\t414.8\t418.1\t464.8\t488.1\t489.1\t485.7\t581.3\t579.7\t526.2\t551.4\t618.6\t628.5\t578.8\t553.3\t481.5\t455.6\t487.9\t507.3\t497.6\t515.4\t510.2\t490.5\t500.5\t494.1\t532.9\t506.5\t466.6\t438.0\t385.4\t381.2\t385.9\t351.7\t371.3\t340.8\t320.2\t277.0\t228.9\t179.5]"  InternalRulePriority=Speed  RndMeth=Simplest  InputSameDT=on
  Magnitude-Angle to Complex1 : MagnitudeAngleToComplex
  Snubber3 : powerlib/Elements/Series RLC Branch  LConnTagsString=__new0  RConnTagsString=__new0  BranchType=R  Resistance=1e6  Inductance=1e-3  SetiL0=off  InitialCurrent=0  Capacitance=1e-6  Setx0=off  InitialVoltage=0  Measurements=None
      settings: SourceProductName=Simscape Electrical
  meas cur2 : powerlib/Measurements/Current Measurement  PhasorSimulation=on  OutputType=Complex  PSBequivalent=0
      settings: SourceProductName=Simscape Electrical
  Conn1 : PMIOPort  Side=Left
  Conn2 : PMIOPort  Port=2  Side=Right
  Out1 : Outport
  wires:
  meas cur2/1 -> Out1/1
  Clock/1 -> Load Data 1-D Lookup Table/1
  Magnitude-Angle to Complex1/1 -> Controlled Current Source4/1
  Load Data 1-D Lookup Table/1 -> Gain6/1
  Complex to Magnitude-Angle/1 -> Magnitude-Angle to Complex1/2
  Gain10/1 -> Magnitude-Angle to Complex1/1
  Gain6/1 -> Gain10/1
  [Vsec] -> Complex to Magnitude-Angle/1
  connections:
  Conn1/RConn1 -- meas cur2/LConn1
  Snubber3/LConn1 -- meas cur2/RConn1 -- Controlled Current Source4/RConn1
  Snubber3/RConn1 -- Controlled Current Source4/LConn1 -- Conn2/RConn1

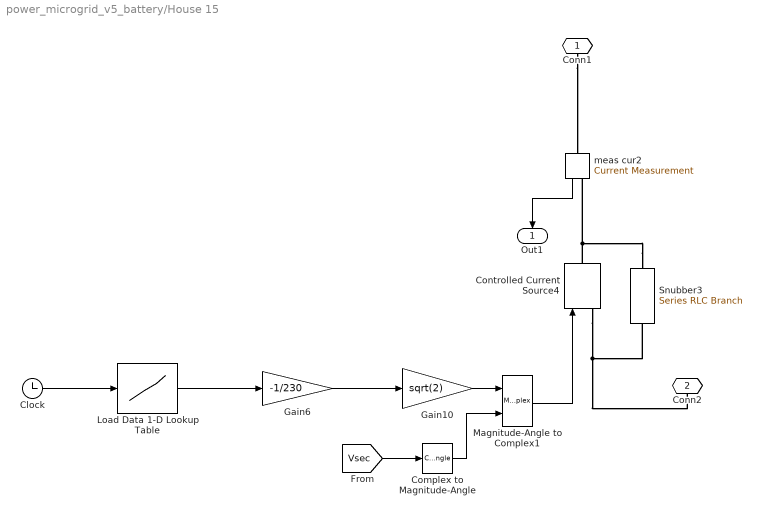
== system power_microgrid_v5_battery/House 15 ==
  Clock : Clock
  Complex to Magnitude-Angle : ComplexToMagnitudeAngle  Output=Angle
  Controlled Current Source4 : powerlib/Electrical Sources/Controlled Current Source  Initialize=on  Source_Type=AC  Amplitude=0  Phase=0  Frequency=50  Measurements=None
      settings: SourceProductName=Simscape Electrical
  Gain10 : Gain  Gain=sqrt(2)
  Gain6 : Gain  Gain=-1/230
  Load Data 1-D Lookup Table : Lookup_n-D  NumberOfTableDimensions=1  BreakpointsForDimension1="[0.00\t600.00\t1200.00\t1800.00\t2400.00\t3000.00\t3600.00\t4200.00\t4800.00\t5400.00\t6000.00\t6600.00\t7200.00\t7800.00\t8400.00\t9000.00\t9600.00\t10200.00\t10800.00\t11400.00\t12000.00\t12600.00\t13200.00\t13800.00\t14400.00\t15000.00\t15600.00\t16200.00\t16800.00\t17400.00\t18000.00\t18600.00\t19200.00\t19800.00\t20400.00\t21000.00\t21600.00\t22200.00\t22800.00\t23400.00\t24000.00\t24600.00\t25200.00\t25800.00\t26400.00\t27000.00\t27600.00\t28200.00\t28800.00\t29400.00\t30000.00\t30600.00\t31200.00\t31800.00\t32400.00\t33000.00\t33600.00\t34200.00\t34800.00\t35400.00\t36000.00\t36600.00\t37200.00\t37800.00\t38400.00\t39000.00\t39600.00\t40200.00\t40800.00\t41400.00\t42000.00\t42600.00\t43200.00\t43800.00\t44400.00\t45000.00\t45600.00\t46200.00\t46800.00\t47400.00\t48000.00\t48600.00\t49200.00\t49800.00\t50400.00\t51000.00\t51600.00\t52200.00\t52800.00\t53400.00\t54000.00\t54600.00\t55200.00\t55800.00\t56400.00\t57000.00\t57600.00\t58200.00\t58800.00\t59400.00\t60000.00\t60600.00\t61200.00\t61800.00\t62400.00\t63000.00\t63600.00\t64200.00\t64800.00\t65400.00\t66000.00\t66600.00\t67200.00\t67800.00\t68400.00\t69000.00\t69600.00\t70200.00\t70800.00\t71400.00\t72000.00\t72600.00\t73200.00\t73800.00\t74400.00\t75000.00\t75600.00\t76200.00\t76800.00\t77400.00\t78000.00\t78600.00\t79200.00\t79800.00\t80400.00\t81000.00\t81600.00\t82200.00\t82800.00\t83400.00\t84000.00\t84600.00\t85200.00\t85800.00\t86400.00]"  BeginIndexSearchUsingPreviousIndexResult=on  Table="[179.5\t163.3\t152.9\t132.5\t118.9\t111.3\t124.6\t103.3\t83.5\t81.2\t85.9\t85.2\t91.9\t95.6\t95.9\t81.8\t83.7\t86.7\t93.8\t81.2\t92.7\t99.4\t112.6\t88.2\t85.6\t78.4\t88.4\t93.9\t86.1\t86.0\t111.7\t143.5\t122.7\t136.8\t142.2\t135.1\t145.6\t141.8\t152.1\t140.3\t167.9\t256.6\t226.1\t263.8\t283.9\t303.3\t279.5\t294.9\t282.3\t288.8\t333.5\t360.9\t421.4\t494.2\t392.5\t439.7\t395.9\t394.4\t364.9\t353.0\t359.1\t370.9\t398.5\t447.4\t344.5\t330.8\t306.8\t331.3\t331.9\t307.6\t371.3\t387.4\t376.6\t360.2\t414.1\t445.1\t411.1\t389.5\t425.2\t340.0\t316.3\t332.8\t352.3\t301.8\t261.8\t298.1\t350.9\t327.8\t296.5\t319.6\t368.4\t327.2\t265.7\t277.9\t292.9\t301.4\t377.9\t336.0\t324.6\t353.8\t389.7\t355.9\t328.4\t325.9\t378.1\t338.0\t379.1\t414.8\t418.1\t464.8\t488.1\t489.1\t485.7\t581.3\t579.7\t526.2\t551.4\t618.6\t628.5\t578.8\t553.3\t481.5\t455.6\t487.9\t507.3\t497.6\t515.4\t510.2\t490.5\t500.5\t494.1\t532.9\t506.5\t466.6\t438.0\t385.4\t381.2\t385.9\t351.7\t371.3\t340.8\t320.2\t277.0\t228.9\t179.5]"  InternalRulePriority=Speed  RndMeth=Simplest  InputSameDT=on
  Magnitude-Angle to Complex1 : MagnitudeAngleToComplex
  Snubber3 : powerlib/Elements/Series RLC Branch  LConnTagsString=__new0  RConnTagsString=__new0  BranchType=R  Resistance=1e6  Inductance=1e-3  SetiL0=off  InitialCurrent=0  Capacitance=1e-6  Setx0=off  InitialVoltage=0  Measurements=None
      settings: SourceProductName=Simscape Electrical
  meas cur2 : powerlib/Measurements/Current Measurement  PhasorSimulation=on  OutputType=Complex  PSBequivalent=0
      settings: SourceProductName=Simscape Electrical
  Conn1 : PMIOPort  Side=Left
  Conn2 : PMIOPort  Port=2  Side=Right
  Out1 : Outport
  wires:
  meas cur2/1 -> Out1/1
  Clock/1 -> Load Data 1-D Lookup Table/1
  Magnitude-Angle to Complex1/1 -> Controlled Current Source4/1
  Load Data 1-D Lookup Table/1 -> Gain6/1
  Complex to Magnitude-Angle/1 -> Magnitude-Angle to Complex1/2
  Gain10/1 -> Magnitude-Angle to Complex1/1
  Gain6/1 -> Gain10/1
  [Vsec] -> Complex to Magnitude-Angle/1
  connections:
  Conn1/RConn1 -- meas cur2/LConn1
  Snubber3/LConn1 -- meas cur2/RConn1 -- Controlled Current Source4/RConn1
  Snubber3/RConn1 -- Controlled Current Source4/LConn1 -- Conn2/RConn1
